simulink model "Question_1"  (R2024b)
settings: Solver=VariableStepAuto  StartTime=0.0  StopTime=10.0  RelTol=1e-3
model workspace (MAT data in the model file):
  F = 100
  M = 100
  b = 50
  k = 100
settings Model: Creator=Sagar  LastModifiedBy=Sagar

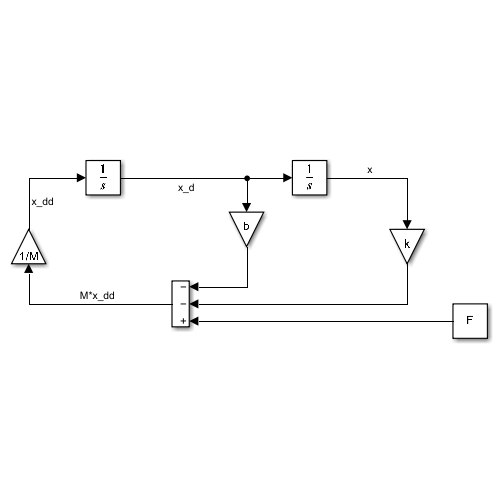
[thumbnail: Simulink's stored preview of the top-level diagram]
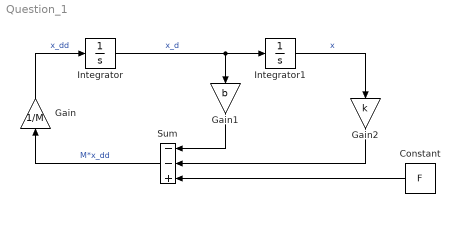
== system Question_1 ==
  Constant : Constant  Value=F
  Gain : Gain  Gain=1/M
  Gain1 : Gain  Gain=b
  Gain2 : Gain  Gain=k
  Integrator : Integrator
  Integrator1 : Integrator
  Sum : Sum  Inputs=--+
  wires:
  Gain/1 -> Integrator/1  "x_dd"
  Integrator/1 -> Integrator1/1, Gain1/1  "x_d"
  Integrator1/1 -> Gain2/1  "x"
  Gain2/1 -> Sum/2
  Sum/1 -> Gain/1  "M*x_dd"
  Gain1/1 -> Sum/1
  Constant/1 -> Sum/3
